simulink model "Lab7_E1"  (R2020b)
settings: Solver=VariableStepAuto  StartTime=0.0  StopTime=10  FixedStep=0  RelTol=1e-3
libraries: neural x28, simulink x2
(part 1 of 2)
settings Model: Creator=smsmt  LastModifiedBy=smsmt

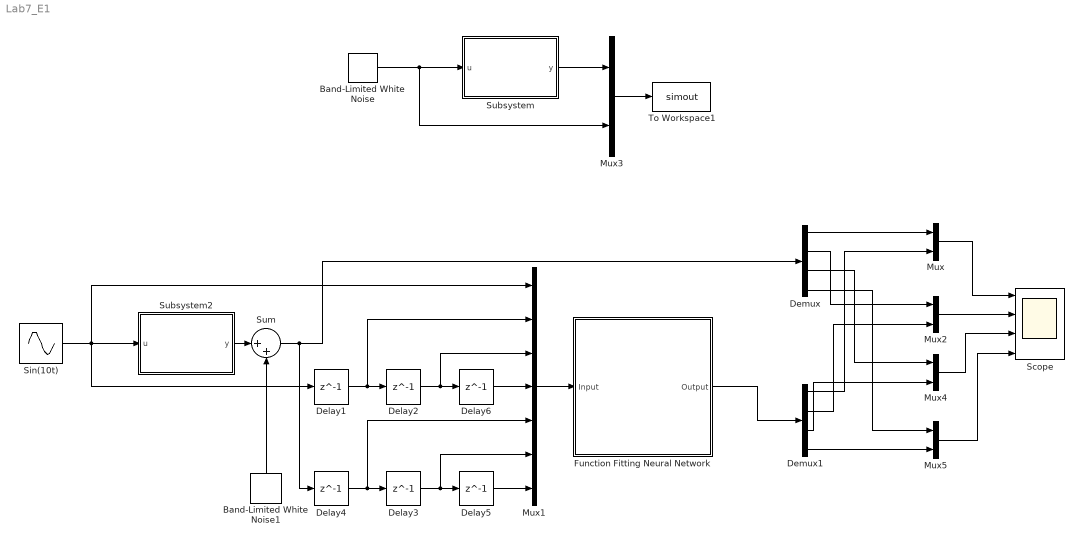
== system Lab7_E1 ==
  Band-Limited White Noise : simulink/Sources/Band-Limited White Noise  Cov=[0.1]  Ts=0.1  seed=[23341]
  Band-Limited White Noise1 : simulink/Sources/Band-Limited White Noise  Cov=[0.000]  Ts=0.1  seed=[23341]
  Delay{1..6} (6 alike) : Delay  DelayLength=1  InitialCondition=0
  Demux : Demux
  Demux1 : Demux
  Function Fitting Neural Network : Subsystem
      mask help: Function Fitting Neural Network
      mask Display: e = 0.06;c1 = [120 150 230]/255;c2 = ([120 150 230]+0)/383;c3 = ([120 150 230]+128)/383;patch([0 1 1 0],[0 0 1 1],c1);patch([0 1 1 1-e 1-e 0+e],[0 0 1 1-e 0+e 0+e],c2);patch([0 0 1 1-e 0+e 0+e],[0 1 1 1-e 1-e 0+e],c3);plot([0 1 1 0 0],[0 0 1 1 0]);fprintf('NNET');port_label('input',1,' Input');port_label('output',1,'Output ');
  Mux{,2..5} (5 alike) : Mux  Inputs=2
  Mux1 : Mux  Inputs=7
  Scope : Scope  NumInputPorts=4
  Sin(10t) : Sin  Frequency=10  SampleTime=0
  Subsystem : Subsystem
  Subsystem2 : Subsystem
  Sum : Sum  Inputs=|++
  To Workspace1 : ToWorkspace  VariableName=simout  SaveFormat=Timeseries  SampleTime=-1
  wires:
  Delay1/1 -> Mux1/2, Delay2/1
  Delay6/1 -> Mux1/4
  Delay4/1 -> Mux1/5, Delay3/1
  Mux1/1 -> Function Fitting Neural Network/1(Input)
  Delay5/1 -> Mux1/7
  Sin(10t)/1 -> Mux1/1, Delay1/1, Subsystem2/1(u)
  Subsystem2/1(y) -> Sum/1
  Delay2/1 -> Mux1/3, Delay6/1
  Delay3/1 -> Mux1/6, Delay5/1
  Mux3/1 -> To Workspace1/1
  Band-Limited White Noise/1 -> Subsystem/1(u), Mux3/2
  Subsystem/1(y) -> Mux3/1
  Function Fitting Neural Network/1(Output) -> Demux1/1
  Demux/1 -> Mux/1
  Demux1/1 -> Mux/2
  Mux/1 -> Scope/1
  Demux/2 -> Mux2/1
  Demux1/2 -> Mux2/2
  Demux/3 -> Mux4/1
  Demux1/3 -> Mux4/2
  Demux/4 -> Mux5/1
  Demux1/4 -> Mux5/2
  Mux5/1 -> Scope/4
  Mux4/1 -> Scope/3
  Mux2/1 -> Scope/2
  Sum/1 -> Delay4/1, Demux/1
  Band-Limited White Noise1/1 -> Sum/2

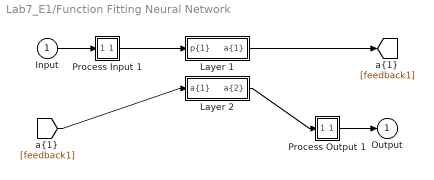
== system Lab7_E1/Function Fitting Neural Network ==
  Input : Inport  PortDimensions=16
      mask Display: e = 0.06;c1 = [120 230 180]/255;c2 = ([120 230 180]+0)/(256+128);c3 = ([120 230 180]+128)/(256+128);patch([0 1 1 0],[0 0 1 1],c1);patch([0 1 1 1-e 1-e 0+e],[0 0 1 1-e 0+e 0+e],c2);patch([0 0 1 1-e 0+e 0+e],[0 1 1 1-e 1-e 0+e],c3);plot([0 1 1 0 0],[0 0 1 1 0]);
  Layer 1 : Subsystem
      mask Display: e = 0.06;c1 = [120 150 230]/255;c2 = ([120 150 230]+0)/383;c3 = ([120 150 230]+128)/383;patch([0 1 1 0],[0 0 1 1],c1);patch([0 1 1 1-e 1-e 0+e],[0 0 1 1-e 0+e 0+e],c2);patch([0 0 1 1-e 0+e 0+e],[0 1 1 1-e 1-e 0+e],c3);plot([0 1 1 0 0],[0 0 1 1 0]);
  Layer 2 : Subsystem
      mask Display: e = 0.06;c1 = [120 150 230]/255;c2 = ([120 150 230]+0)/383;c3 = ([120 150 230]+128)/383;patch([0 1 1 0],[0 0 1 1],c1);patch([0 1 1 1-e 1-e 0+e],[0 0 1 1-e 0+e 0+e],c2);patch([0 0 1 1-e 0+e 0+e],[0 1 1 1-e 1-e 0+e],c3);plot([0 1 1 0 0],[0 0 1 1 0]);
  Process Input 1 : Subsystem
      mask Display: e = 0.06;c1 = [120 150 230]/255;c2 = ([120 150 230]+0)/383;c3 = ([120 150 230]+128)/383;patch([0 1 1 0],[0 0 1 1],c1);patch([0 1 1 1-e 1-e 0+e],[0 0 1 1-e 0+e 0+e],c2);patch([0 0 1 1-e 0+e 0+e],[0 1 1 1-e 1-e 0+e],c3);plot([0 1 1 0 0],[0 0 1 1 0]);
  Process Output 1 : Subsystem
      mask Display: e = 0.06;c1 = [120 150 230]/255;c2 = ([120 150 230]+0)/383;c3 = ([120 150 230]+128)/383;patch([0 1 1 0],[0 0 1 1],c1);patch([0 1 1 1-e 1-e 0+e],[0 0 1 1-e 0+e 0+e],c2);patch([0 0 1 1-e 0+e 0+e],[0 1 1 1-e 1-e 0+e],c3);plot([0 1 1 0 0],[0 0 1 1 0]);
  Output : Outport  InitialOutput=[0;0;0;0]
      mask Display: e = 0.06;c1 = [120 230 180]/255;c2 = ([120 230 180]+0)/(256+128);c3 = ([120 230 180]+128)/(256+128);patch([0 1 1 0],[0 0 1 1],c1);patch([0 1 1 1-e 1-e 0+e],[0 0 1 1-e 0+e 0+e],c2);patch([0 0 1 1-e 0+e 0+e],[0 1 1 1-e 1-e 0+e],c3);plot([0 1 1 0 0],[0 0 1 1 0]);
  wires:
  Input/1 -> Process Input 1/1(x)
  Process Output 1/1(y) -> Output/1
  Process Input 1/1(p) -> Layer 1/1("p{1}")
  Layer 1/1("a{1}") -> [feedback1]
  [feedback1] -> Layer 2/1("a{1} ")
  Layer 2/1("a{2}") -> Process Output 1/1(a)

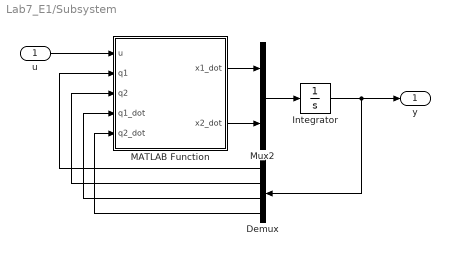
== system Lab7_E1/Subsystem ==
  u : Inport
  Demux : Demux
  Integrator : Integrator  InitialCondition=[0 0 0 0]
  MATLAB Function : MATLAB Function  TreatAsAtomicUnit=on
  Mux2 : Mux  Inputs=2
  y : Outport
  wires:
  Integrator/1 -> y/1, Demux/1
  u/1 -> MATLAB Function/1(u)
  MATLAB Function/1(x1_dot) -> Mux2/1
  MATLAB Function/2(x2_dot) -> Mux2/2
  Mux2/1 -> Integrator/1
  Demux/1 -> MATLAB Function/2(q1)
  Demux/2 -> MATLAB Function/3(q2)
  Demux/3 -> MATLAB Function/4(q1_dot)
  Demux/4 -> MATLAB Function/5(q2_dot)

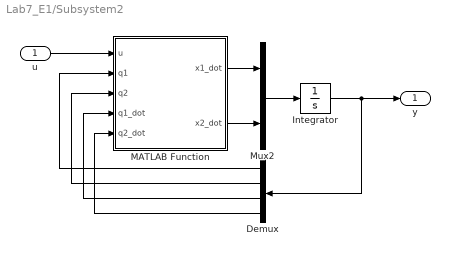
== system Lab7_E1/Subsystem2 ==
  u : Inport
  Demux : Demux
  Integrator : Integrator  InitialCondition=[0 0 0 0]
  MATLAB Function : MATLAB Function  TreatAsAtomicUnit=on
  Mux2 : Mux  Inputs=2
  y : Outport
  wires:
  Integrator/1 -> y/1, Demux/1
  u/1 -> MATLAB Function/1(u)
  MATLAB Function/1(x1_dot) -> Mux2/1
  MATLAB Function/2(x2_dot) -> Mux2/2
  Mux2/1 -> Integrator/1
  Demux/1 -> MATLAB Function/2(q1)
  Demux/2 -> MATLAB Function/3(q2)
  Demux/3 -> MATLAB Function/4(q1_dot)
  Demux/4 -> MATLAB Function/5(q2_dot)

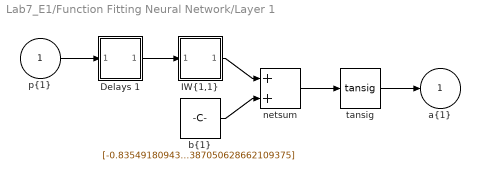
== system Lab7_E1/Function Fitting Neural Network/Layer 1 ==
  "p{1}" : Inport  PortDimensions=16
      mask Display: e = 0.06;c1 = [120 230 180]/255;c2 = ([120 230 180]+0)/(256+128);c3 = ([120 230 180]+128)/(256+128);patch([0 1 1 0],[0 0 1 1],c1);patch([0 1 1 1-e 1-e 0+e],[0 0 1 1-e 0+e 0+e],c2);patch([0 0 1 1-e 0+e 0+e],[0 1 1 1-e 1-e 0+e],c3);plot([0 1 1 0 0],[0 0 1 1 0]);
  Delays 1 : Subsystem
      mask Display: e = 0.06;c1 = [120 150 230]/255;c2 = ([120 150 230]+0)/383;c3 = ([120 150 230]+128)/383;patch([0 1 1 0],[0 0 1 1],c1);patch([0 1 1 1-e 1-e 0+e],[0 0 1 1-e 0+e 0+e],c2);patch([0 0 1 1-e 0+e 0+e],[0 1 1 1-e 1-e 0+e],c3);plot([0 1 1 0 0],[0 0 1 1 0]);disp('0');
  "IW{1,1}" : Subsystem
      mask Display: e = 0.06;c1 = [120 150 230]/255;c2 = ([120 150 230]+0)/383;c3 = ([120 150 230]+128)/383;patch([0 1 1 0],[0 0 1 1],c1);patch([0 1 1 1-e 1-e 0+e],[0 0 1 1-e 0+e 0+e],c2);patch([0 0 1 1-e 0+e 0+e],[0 1 1 1-e 1-e 0+e],c3);plot([0 1 1 0 0],[0 0 1 1 0]);disp('W');
  "b{1}" : Constant  Value=[-0.83549180943357848061481263357563875615596771240234375;-1.8201004242661380505552415343117900192737579345703125;0.92350959078641003952014898459310643374919891357421875;-0.92781891823089457371764865456498228013515472412109375;-0.98835326541109835840615005508880130946636199951171875;0.94440562253181947749425262372824363410472869873046875;-0.0199942887878296442216718986628620768897235393524169921875;-0.5282206006504706063964249551645480096340179443359375;-0.306513926556519933352973339424352161586284637451171875;0.00887448769022419238494681081874659867025911808013916015625;0.10503960517018810782996496300256694667041301727294921875;0.363930984793109202346528263660729862749576568603515625;0.853259192692973567062608708511106669902801513671875;-0.479073523910536536174475941152195446193218231201171875;0.386311529121468211211976040431181900203227996826171875;-0.50019372501267433950289387212251313030719757080078125;-0.84925071198815149653427170051145367324352264404296875;0.330688290295932219020613729298929683864116668701171875;1.0433757247374746413015600410290062427520751953125;1.810341107309246577727890326059423387050628662109375]
      mask Display: e = 0.06;c1 = [120 150 230]/255;c2 = ([120 150 230]+0)/383;c3 = ([120 150 230]+128)/383;patch([0 1 1 0],[0 0 1 1],c1);patch([0 1 1 1-e 1-e 0+e],[0 0 1 1-e 0+e 0+e],c2);patch([0 0 1 1-e 0+e 0+e],[0 1 1 1-e 1-e 0+e],c3);plot([0 1 1 0 0],[0 0 1 1 0]);disp('b');
  netsum : Sum  Inputs=2  InputSameDT=on  SaturateOnIntegerOverflow=on  OutDataTypeStr=Inherit: Same as first input
      mask Display: e = 0.06;c1 = [120 150 230]/255;c2 = ([120 150 230]+0)/383;c3 = ([120 150 230]+128)/383;patch([0 1 1 0],[0 0 1 1],c1);patch([0 1 1 1-e 1-e 0+e],[0 0 1 1-e 0+e 0+e],c2);patch([0 0 1 1-e 0+e 0+e],[0 1 1 1-e 1-e 0+e],c3);plot([0 1 1 0 0],[0 0 1 1 0]);disp('+');
  tansig : neural/Transfer Functions/tansig
  "a{1}" : Outport  InitialOutput=[0;0;0;0;0;0;0;0;0;0;0;0;0;0;0;0;0;0;0;0]
      mask Display: e = 0.06;c1 = [120 230 180]/255;c2 = ([120 230 180]+0)/(256+128);c3 = ([120 230 180]+128)/(256+128);patch([0 1 1 0],[0 0 1 1],c1);patch([0 1 1 1-e 1-e 0+e],[0 0 1 1-e 0+e 0+e],c2);patch([0 0 1 1-e 0+e 0+e],[0 1 1 1-e 1-e 0+e],c3);plot([0 1 1 0 0],[0 0 1 1 0]);
  wires:
  "p{1}"/1 -> Delays 1/1("p{1}")
  Delays 1/1("pd{1,1}") -> "IW{1,1}"/1("pd{1,1}")
  "IW{1,1}"/1("iz{1,1}") -> netsum/1
  "b{1}"/1 -> netsum/2
  netsum/1 -> tansig/1
  tansig/1 -> "a{1}"/1

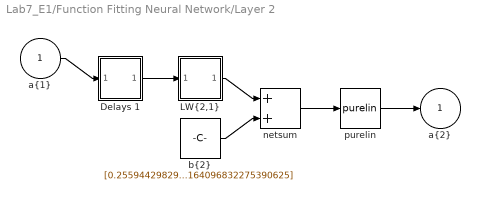
== system Lab7_E1/Function Fitting Neural Network/Layer 2 ==
  "a{1} " : Inport  PortDimensions=20
      mask Display: e = 0.06;c1 = [120 230 180]/255;c2 = ([120 230 180]+0)/(256+128);c3 = ([120 230 180]+128)/(256+128);patch([0 1 1 0],[0 0 1 1],c1);patch([0 1 1 1-e 1-e 0+e],[0 0 1 1-e 0+e 0+e],c2);patch([0 0 1 1-e 0+e 0+e],[0 1 1 1-e 1-e 0+e],c3);plot([0 1 1 0 0],[0 0 1 1 0]);
  Delays 1 : Subsystem
      mask Display: e = 0.06;c1 = [120 150 230]/255;c2 = ([120 150 230]+0)/383;c3 = ([120 150 230]+128)/383;patch([0 1 1 0],[0 0 1 1],c1);patch([0 1 1 1-e 1-e 0+e],[0 0 1 1-e 0+e 0+e],c2);patch([0 0 1 1-e 0+e 0+e],[0 1 1 1-e 1-e 0+e],c3);plot([0 1 1 0 0],[0 0 1 1 0]);disp('0');
  "LW{2,1}" : Subsystem
      mask Display: e = 0.06;c1 = [120 150 230]/255;c2 = ([120 150 230]+0)/383;c3 = ([120 150 230]+128)/383;patch([0 1 1 0],[0 0 1 1],c1);patch([0 1 1 1-e 1-e 0+e],[0 0 1 1-e 0+e 0+e],c2);patch([0 0 1 1-e 0+e 0+e],[0 1 1 1-e 1-e 0+e],c3);plot([0 1 1 0 0],[0 0 1 1 0]);disp('W');
  "b{2}" : Constant  Value=[0.25594429829992548786066208776901476085186004638671875;0.10194009318987629075792256116983480751514434814453125;0.55700857727010311126747410526149906218051910400390625;0.1142790231718998905652284747702651657164096832275390625]
      mask Display: e = 0.06;c1 = [120 150 230]/255;c2 = ([120 150 230]+0)/383;c3 = ([120 150 230]+128)/383;patch([0 1 1 0],[0 0 1 1],c1);patch([0 1 1 1-e 1-e 0+e],[0 0 1 1-e 0+e 0+e],c2);patch([0 0 1 1-e 0+e 0+e],[0 1 1 1-e 1-e 0+e],c3);plot([0 1 1 0 0],[0 0 1 1 0]);disp('b');
  netsum : Sum  Inputs=2  InputSameDT=on  SaturateOnIntegerOverflow=on  OutDataTypeStr=Inherit: Same as first input
      mask Display: e = 0.06;c1 = [120 150 230]/255;c2 = ([120 150 230]+0)/383;c3 = ([120 150 230]+128)/383;patch([0 1 1 0],[0 0 1 1],c1);patch([0 1 1 1-e 1-e 0+e],[0 0 1 1-e 0+e 0+e],c2);patch([0 0 1 1-e 0+e 0+e],[0 1 1 1-e 1-e 0+e],c3);plot([0 1 1 0 0],[0 0 1 1 0]);disp('+');
  purelin : neural/Transfer Functions/purelin
  "a{2}" : Outport  InitialOutput=[0;0;0;0]
      mask Display: e = 0.06;c1 = [120 230 180]/255;c2 = ([120 230 180]+0)/(256+128);c3 = ([120 230 180]+128)/(256+128);patch([0 1 1 0],[0 0 1 1],c1);patch([0 1 1 1-e 1-e 0+e],[0 0 1 1-e 0+e 0+e],c2);patch([0 0 1 1-e 0+e 0+e],[0 1 1 1-e 1-e 0+e],c3);plot([0 1 1 0 0],[0 0 1 1 0]);
  wires:
  "a{1} "/1 -> Delays 1/1("p{2}")
  Delays 1/1("pd{2,1}") -> "LW{2,1}"/1("ad{2,1}")
  "LW{2,1}"/1("lz{2,1}") -> netsum/1
  "b{2}"/1 -> netsum/2
  netsum/1 -> purelin/1
  purelin/1 -> "a{2}"/1

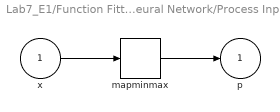
== system Lab7_E1/Function Fitting Neural Network/Process Input 1 ==
  x : Inport  PortDimensions=16
      mask Display: e = 0.06;c1 = [120 230 180]/255;c2 = ([120 230 180]+0)/(256+128);c3 = ([120 230 180]+128)/(256+128);patch([0 1 1 0],[0 0 1 1],c1);patch([0 1 1 1-e 1-e 0+e],[0 0 1 1-e 0+e 0+e],c2);patch([0 0 1 1-e 0+e 0+e],[0 1 1 1-e 1-e 0+e],c3);plot([0 1 1 0 0],[0 0 1 1 0]);
  mapminmax : neural/Processing Functions/mapminmax  xmin=[-3.60517824283159749043647934741;-3.60517824283159749043647934741;-3.60517824283159749043647934741;-3.60517824283159749043647934741;-3.14106589513792666679137255414;-0.492448062530743690956569480477;-2.84100174011369333015863958281;-0.745389047564771978215958370129;-3.14106589513792666679137255414;-0.492448062530743690956569480477;-2.84100174011369333015863958281;-0.745389047564771978215958370129;-3.14106589513792666679137255414;-0.492448062530743690956569480477;-2.84100174011369333015863958281;-0.745389047564771978215958370129]  xmax=[3.94389172900844897640126873739;3.94389172900844897640126873739;3.94389172900844897640126873739;3.94389172900844897640126873739;0.0005725595982868994515690985736;0.491232002437546833029102799628;2.83941327458839021247172240692;0.745062684061230662280195247149;0.0005725595982868994515690985736;0.491232002437546833029102799628;2.83941327458839021247172240692;0.745062684061230662280195247149;0.0005725595982868994515690985736;0.491232002437546833029102799628;2.83941327458839021247172240692;0.745062684061230662280195247149]  ymin=-1  ymax=1
  p : Outport  PortDimensions=16
      mask Display: e = 0.06;c1 = [120 230 180]/255;c2 = ([120 230 180]+0)/(256+128);c3 = ([120 230 180]+128)/(256+128);patch([0 1 1 0],[0 0 1 1],c1);patch([0 1 1 1-e 1-e 0+e],[0 0 1 1-e 0+e 0+e],c2);patch([0 0 1 1-e 0+e 0+e],[0 1 1 1-e 1-e 0+e],c3);plot([0 1 1 0 0],[0 0 1 1 0]);
  wires:
  x/1 -> mapminmax/1
  mapminmax/1 -> p/1

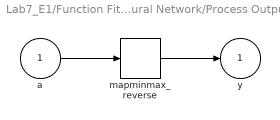
== system Lab7_E1/Function Fitting Neural Network/Process Output 1 ==
  a : Inport  PortDimensions=4
      mask Display: e = 0.06;c1 = [120 230 180]/255;c2 = ([120 230 180]+0)/(256+128);c3 = ([120 230 180]+128)/(256+128);patch([0 1 1 0],[0 0 1 1],c1);patch([0 1 1 1-e 1-e 0+e],[0 0 1 1-e 0+e 0+e],c2);patch([0 0 1 1-e 0+e 0+e],[0 1 1 1-e 1-e 0+e],c3);plot([0 1 1 0 0],[0 0 1 1 0]);
  mapminmax_reverse : neural/Processing Functions/mapminmax_reverse  xmin=[-3.14106589513792666679137255414;-0.492448062530743690956569480477;-2.84100174011369333015863958281;-0.745389047564771978215958370129]  xmax=[0.0005725595982868994515690985736;0.491232002437546833029102799628;2.83941327458839021247172240692;0.745062684061230662280195247149]  ymin=-1  ymax=1
  y : Outport  PortDimensions=4
      mask Display: e = 0.06;c1 = [120 230 180]/255;c2 = ([120 230 180]+0)/(256+128);c3 = ([120 230 180]+128)/(256+128);patch([0 1 1 0],[0 0 1 1],c1);patch([0 1 1 1-e 1-e 0+e],[0 0 1 1-e 0+e 0+e],c2);patch([0 0 1 1-e 0+e 0+e],[0 1 1 1-e 1-e 0+e],c3);plot([0 1 1 0 0],[0 0 1 1 0]);
  wires:
  a/1 -> mapminmax_reverse/1
  mapminmax_reverse/1 -> y/1

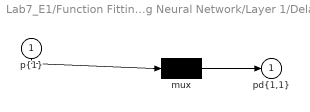
== system Lab7_E1/Function Fitting Neural Network/Layer 1/Delays 1 ==
  "p{1}" : Inport  PortDimensions=16
      mask Display: e = 0.06;c1 = [120 230 180]/255;c2 = ([120 230 180]+0)/(256+128);c3 = ([120 230 180]+128)/(256+128);patch([0 1 1 0],[0 0 1 1],c1);patch([0 1 1 1-e 1-e 0+e],[0 0 1 1-e 0+e 0+e],c2);patch([0 0 1 1-e 0+e 0+e],[0 1 1 1-e 1-e 0+e],c3);plot([0 1 1 0 0],[0 0 1 1 0]);
  mux : Mux  Inputs=1
      mask Display: e = 0.06;c1 = [120 150 230]/255;c2 = ([120 150 230]+0)/383;c3 = ([120 150 230]+128)/383;patch([0 1 1 0],[0 0 1 1],c1);patch([0 1 1 1-e 1-e 0+e],[0 0 1 1-e 0+e 0+e],c2);patch([0 0 1 1-e 0+e 0+e],[0 1 1 1-e 1-e 0+e],c3);plot([0 1 1 0 0],[0 0 1 1 0]);disp('Mux')
  "pd{1,1}" : Outport
      mask Display: e = 0.06;c1 = [120 230 180]/255;c2 = ([120 230 180]+0)/(256+128);c3 = ([120 230 180]+128)/(256+128);patch([0 1 1 0],[0 0 1 1],c1);patch([0 1 1 1-e 1-e 0+e],[0 0 1 1-e 0+e 0+e],c2);patch([0 0 1 1-e 0+e 0+e],[0 1 1 1-e 1-e 0+e],c3);plot([0 1 1 0 0],[0 0 1 1 0]);
  wires:
  "p{1}"/1 -> mux/1
  mux/1 -> "pd{1,1}"/1

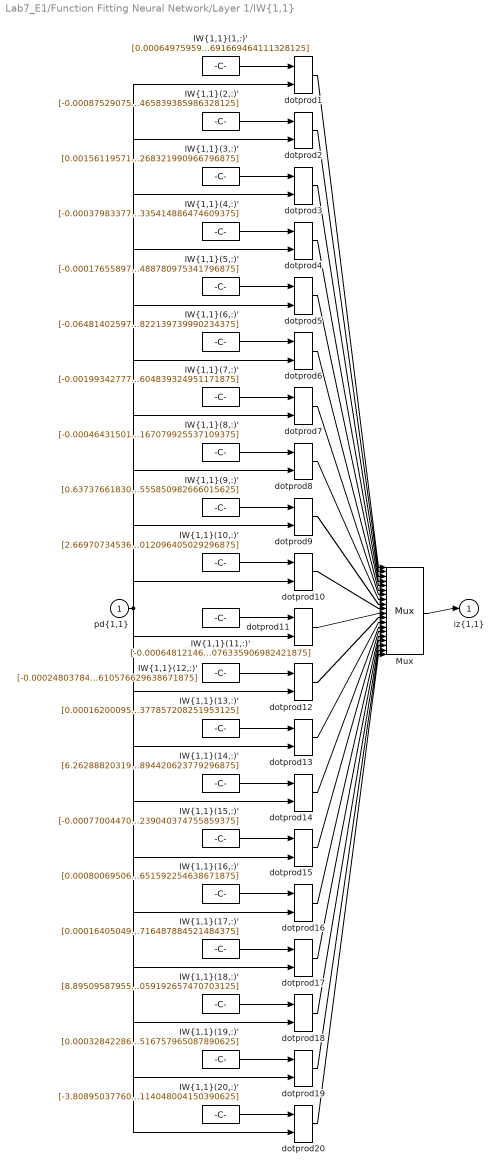
== system Lab7_E1/Function Fitting Neural Network/Layer 1/IW{1,1} ==
  "pd{1,1}" : Inport  PortDimensions=16
      mask Display: e = 0.06;c1 = [120 230 180]/255;c2 = ([120 230 180]+0)/(256+128);c3 = ([120 230 180]+128)/(256+128);patch([0 1 1 0],[0 0 1 1],c1);patch([0 1 1 1-e 1-e 0+e],[0 0 1 1-e 0+e 0+e],c2);patch([0 0 1 1-e 0+e 0+e],[0 1 1 1-e 1-e 0+e],c3);plot([0 1 1 0 0],[0 0 1 1 0]);
  "IW{1,1}(1,:)'" : Constant  Value=[0.0006497595962778571383744452560904392157681286334991455078125;-4.14681874647082770080248892430319074264843948185443878173828125e-05;-0.000117323732129381670869806841839277922190376557409763336181640625;-0.00081712479590169829861412420513033794122748076915740966796875;0.02054128798901501407048186820247792638838291168212890625;-0.222381987091993471583606378771946765482425689697265625;-0.08351944219501715449549550385199836455285549163818359375;-0.012355659297301264942792187184750218875706195831298828125;0.435902112701866517596727135241962969303131103515625;0.319137008096920304911492394239758141338825225830078125;0.1420357879260343292315837970818392932415008544921875;0.059008653478310912898763263001455925405025482177734375;-0.472592024618235073685212910277186892926692962646484375;-0.48057038845304023144677785239764489233493804931640625;-0.1660689221136188165051095211310894228518009185791015625;-0.1158794303381847357048428648340632207691669464111328125]
      mask Display: e = 0.06;c1 = [120 150 230]/255;c2 = ([120 150 230]+0)/383;c3 = ([120 150 230]+128)/383;patch([0 1 1 0],[0 0 1 1],c1);patch([0 1 1 1-e 1-e 0+e],[0 0 1 1-e 0+e 0+e],c2);patch([0 0 1 1-e 0+e 0+e],[0 1 1 1-e 1-e 0+e],c3);plot([0 1 1 0 0],[0 0 1 1 0]);disp('Weights');
  "IW{1,1}(10,:)'" : Constant  Value=[2.669707345365600827829556662695864588386029936373233795166015625e-05;6.163721756815836064040403652342092755134217441082000732421875e-05;0.00085904376332920592308772800294036642299033701419830322265625;-0.000748848611049175217659057413044365603127516806125640869140625;-0.64749101968490607728057284475653432309627532958984375;0.15628981793171414782506190022104419767856597900390625;0.41368487647578866539532782553578726947307586669921875;-0.25282757750305939747903494208003394305706024169921875;1.8245352517186936847082279200549237430095672607421875;-0.1258491512073245666147869314954732544720172882080078125;0.2105603075066311280494346647174097597599029541015625;0.39732536199083423600342257486772723495960235595703125;-1.1556706822333964179705390051822178065776824951171875;-0.0257373295222910851431930012722659739665687084197998046875;-0.441138402187714107061111690200050361454486846923828125;-0.17624767227669824176672364046680741012096405029296875]
      mask Display: e = 0.06;c1 = [120 150 230]/255;c2 = ([120 150 230]+0)/383;c3 = ([120 150 230]+128)/383;patch([0 1 1 0],[0 0 1 1],c1);patch([0 1 1 1-e 1-e 0+e],[0 0 1 1-e 0+e 0+e],c2);patch([0 0 1 1-e 0+e 0+e],[0 1 1 1-e 1-e 0+e],c3);plot([0 1 1 0 0],[0 0 1 1 0]);disp('Weights');
  "IW{1,1}(11,:)'" : Constant  Value=[-0.000648121461776643707948519779193929934990592300891876220703125;0.000318543579510111897479252007769900956191122531890869140625;0.00125256239143849818461207146214064778177998960018157958984375;-0.00020996056844432974962562366005869307628017850220203399658203125;-0.455149028189702098412539044147706590592861175537109375;0.0192023790503516693373153856327917310409247875213623046875;-0.202090650939533655883195706337573938071727752685546875;-0.1947404938538613572429625264703645370900630950927734375;0.314952753799047246996423154996591620147228240966796875;0.75358597806011273778636905262828804552555084228515625;0.002638631597796150911328094679220157559029757976531982421875;0.440502022320982344893991466960869729518890380859375;-0.2042047006275750364867604957908042706549167633056640625;-0.751880838415297514387702904059551656246185302734375;0.241867536319385789678193532381555996835231781005859375;-0.41794044873874092171917027371819131076335906982421875]
      mask Display: e = 0.06;c1 = [120 150 230]/255;c2 = ([120 150 230]+0)/383;c3 = ([120 150 230]+128)/383;patch([0 1 1 0],[0 0 1 1],c1);patch([0 1 1 1-e 1-e 0+e],[0 0 1 1-e 0+e 0+e],c2);patch([0 0 1 1-e 0+e 0+e],[0 1 1 1-e 1-e 0+e],c3);plot([0 1 1 0 0],[0 0 1 1 0]);disp('Weights');
  "IW{1,1}(12,:)'" : Constant  Value=[-0.0002480378412450206355131798741098236860125325620174407958984375;-0.00020751750405047168887735786757531286639277823269367218017578125;-0.00018989495924129386737223834646925979541265405714511871337890625;0.00034571509970268113516589369993425862048752605915069580078125;-0.11481098550833705729257161465284298174083232879638671875;-0.480672832578880993015246758659486658871173858642578125;0.2005000374408808239135026951771578751504421234130859375;0.00411778208916156567009903000098347547464072704315185546875;0.390440497022451704633994040705147199332714080810546875;0.465074648875374918599590046142111532390117645263671875;-0.5015642578297663245479043325758539140224456787109375;-0.09670273037684502803745800747492467053234577178955078125;-0.50558093037185580786996297320001758635044097900390625;-0.0940046176142029510369724221163778565824031829833984375;0.1497444992321221579612000596171128563582897186279296875;0.07308416151233614044269160103795002214610576629638671875]
      mask Display: e = 0.06;c1 = [120 150 230]/255;c2 = ([120 150 230]+0)/383;c3 = ([120 150 230]+128)/383;patch([0 1 1 0],[0 0 1 1],c1);patch([0 1 1 1-e 1-e 0+e],[0 0 1 1-e 0+e 0+e],c2);patch([0 0 1 1-e 0+e 0+e],[0 1 1 1-e 1-e 0+e],c3);plot([0 1 1 0 0],[0 0 1 1 0]);disp('Weights');
  "IW{1,1}(13,:)'" : Constant  Value=[0.00016200095803150493778931051647163030793308280408382415771484375;0.0003105684530270226323574178639574938642908819019794464111328125;0.000122863321462266385057648943046615386265330016613006591796875;-0.00124550561041928786569499276737360560218803584575653076171875;-0.1692623394344288378920992954590474255383014678955078125;-0.2970496022290927129461124422959983348846435546875;-0.0671470921687993549387130087779951281845569610595703125;0.1399743386114951915200066423494718037545680999755859375;0.50198259880397955168263024461339227855205535888671875;0.2158759395109148548907995746048982255160808563232421875;0.272103660620713616591359595986432395875453948974609375;0.29681257424949947232306612932006828486919403076171875;-0.153500660322007986824388581226230598986148834228515625;0.2078737494795244444834025898671825416386127471923828125;-0.0922669071525324124838363104572636075317859649658203125;-0.217394520222977949419629339899984188377857208251953125]
      mask Display: e = 0.06;c1 = [120 150 230]/255;c2 = ([120 150 230]+0)/383;c3 = ([120 150 230]+128)/383;patch([0 1 1 0],[0 0 1 1],c1);patch([0 1 1 1-e 1-e 0+e],[0 0 1 1-e 0+e 0+e],c2);patch([0 0 1 1-e 0+e 0+e],[0 1 1 1-e 1-e 0+e],c3);plot([0 1 1 0 0],[0 0 1 1 0]);disp('Weights');
  "IW{1,1}(14,:)'" : Constant  Value=[6.26288820319030928827908066836016587330959737300872802734375e-05;0.0003576643112834073582988192452347675498458556830883026123046875;-5.51893240529009778132414620888113176988554187119007110595703125e-05;-8.75221609081757064008133539800837752409279346466064453125e-05;0.779963663071746804433814759249798953533172607421875;0.2936522481223595715249530258006416261196136474609375;-0.418238868048481149397588296778849326074123382568359375;0.13467207616825771498980657270294614136219024658203125;-0.81612352358894046933102117691305465996265411376953125;-0.3477308428804641859954926985665224492549896240234375;0.2216233449633602525796760573939536698162555694580078125;-0.0309948291935520058026920509064439102075994014739990234375;-0.1869254427083924252617208594529074616730213165283203125;0.15814549301092772903842842424637638032436370849609375;-0.1390051880148988894259076687376364134252071380615234375;-0.0095404369545908467020733922936415183357894420623779296875]
      mask Display: e = 0.06;c1 = [120 150 230]/255;c2 = ([120 150 230]+0)/383;c3 = ([120 150 230]+128)/383;patch([0 1 1 0],[0 0 1 1],c1);patch([0 1 1 1-e 1-e 0+e],[0 0 1 1-e 0+e 0+e],c2);patch([0 0 1 1-e 0+e 0+e],[0 1 1 1-e 1-e 0+e],c3);plot([0 1 1 0 0],[0 0 1 1 0]);disp('Weights');
  "IW{1,1}(15,:)'" : Constant  Value=[-0.000770044701256342926758147182653146955999545753002166748046875;-0.000121153238827784843177626239452138179331086575984954833984375;0.000962624329641622732307848497868008053046651184558868408203125;0.001924798690870832031107884318998912931419909000396728515625;1.1900904568608223765835418817005120217800140380859375;-0.1664802091736500011531774134709849022328853607177734375;-0.68768212676038864561434138522599823772907257080078125;-0.250470894826118228859712644407409243285655975341796875;-1.3123900716313710024252259245258755981922149658203125;-0.26442442160472567902473883805214427411556243896484375;0.6451805147554383612629180788644589483737945556640625;-0.051426809903507501864350359710442717187106609344482421875;-0.03580352950115466004188391480056452564895153045654296875;0.294895585737153298477863927473663352429866790771484375;-0.200614027486274382194864074335782788693904876708984375;0.265400607909153762875575921498239040374755859375]
      mask Display: e = 0.06;c1 = [120 150 230]/255;c2 = ([120 150 230]+0)/383;c3 = ([120 150 230]+128)/383;patch([0 1 1 0],[0 0 1 1],c1);patch([0 1 1 1-e 1-e 0+e],[0 0 1 1-e 0+e 0+e],c2);patch([0 0 1 1-e 0+e 0+e],[0 1 1 1-e 1-e 0+e],c3);plot([0 1 1 0 0],[0 0 1 1 0]);disp('Weights');
  "IW{1,1}(16,:)'" : Constant  Value=[0.000800695062533548682602579926737007554038427770137786865234375;-0.00045715830620634352772502229100837212172336876392364501953125;0.0003268933807610846921203051618221024909871630370616912841796875;-5.997773816073786860326999548220783253782428801059722900390625e-05;-0.33597739810910909330488038904150016605854034423828125;0.267747073382606559643903665346442721784114837646484375;-0.57654563164647887330005460171378217637538909912109375;-0.334783999218468297787154597244807519018650054931640625;-0.2065178451448555774216941927079460583627223968505859375;-0.5471426101951986087357227006577886641025543212890625;-0.08439812068263206901175266239079064689576625823974609375;0.10666697974105117385779095684483763761818408966064453125;0.305545296852755388083977550195413641631603240966796875;0.262208114460602492723495515747345052659511566162109375;0.48284509012950216355619659225340001285076141357421875;0.1591205119241236587424026538428734056651592254638671875]
      mask Display: e = 0.06;c1 = [120 150 230]/255;c2 = ([120 150 230]+0)/383;c3 = ([120 150 230]+128)/383;patch([0 1 1 0],[0 0 1 1],c1);patch([0 1 1 1-e 1-e 0+e],[0 0 1 1-e 0+e 0+e],c2);patch([0 0 1 1-e 0+e 0+e],[0 1 1 1-e 1-e 0+e],c3);plot([0 1 1 0 0],[0 0 1 1 0]);disp('Weights');
  "IW{1,1}(17,:)'" : Constant  Value=[0.00016405049724810857707246736225670247222296893596649169921875;-0.0003472694094526647379771178147933596846996806561946868896484375;-0.000858663939336835814637727271048106558737345039844512939453125;1.745347316646612574326906386357194378433632664382457733154296875e-05;-1.669618756525871550167039458756335079669952392578125;-0.65396558716076125250538098043762147426605224609375;1.1620725576523589506194866771693341434001922607421875;0.07796620078256556729545678763315663672983646392822265625;1.3305314701478410110979666569619439542293548583984375;0.0988798833986821168462455489134299568831920623779296875;-1.2198542700796337623359022472868673503398895263671875;-0.0876473476984375443610275624450878240168094635009765625;0.481643337302925356180338667400064878165721893310546875;0.47629794668757530207159334167954511940479278564453125;0.538413625228424397306525861495174467563629150390625;0.08321182076209675260169973398660658858716487884521484375]
      mask Display: e = 0.06;c1 = [120 150 230]/255;c2 = ([120 150 230]+0)/383;c3 = ([120 150 230]+128)/383;patch([0 1 1 0],[0 0 1 1],c1);patch([0 1 1 1-e 1-e 0+e],[0 0 1 1-e 0+e 0+e],c2);patch([0 0 1 1-e 0+e 0+e],[0 1 1 1-e 1-e 0+e],c3);plot([0 1 1 0 0],[0 0 1 1 0]);disp('Weights');
  "IW{1,1}(18,:)'" : Constant  Value=[8.8950958795552698154564252863707451979280449450016021728515625e-05;0.00026509341560794594423733361310269174282439053058624267578125;-0.000403248729956397016470359684348068185499869287014007568359375;0.00142578383093951046971248342032367872889153659343719482421875;-1.3708659490516870160803364342427812516689300537109375;0.10422716158509580386404280716305947862565517425537109375;0.1593468523707887996021526078038732521235942840576171875;0.10771471872017539250787621085692080669105052947998046875;2.0941281483032572197089393739588558673858642578125;0.41506974766941018284427400431013666093349456787109375;0.053450916392035342783461970839198329485952854156494140625;-0.421772112283897160356360700461664237082004547119140625;-0.9212757175698806921815275927656330168247222900390625;-0.56291680190236392800073872422217391431331634521484375;0.0024612492798319189103717352651301553123630583286285400390625;0.26824387557028128714620152095449157059192657470703125]
      mask Display: e = 0.06;c1 = [120 150 230]/255;c2 = ([120 150 230]+0)/383;c3 = ([120 150 230]+128)/383;patch([0 1 1 0],[0 0 1 1],c1);patch([0 1 1 1-e 1-e 0+e],[0 0 1 1-e 0+e 0+e],c2);patch([0 0 1 1-e 0+e 0+e],[0 1 1 1-e 1-e 0+e],c3);plot([0 1 1 0 0],[0 0 1 1 0]);disp('Weights');
  "IW{1,1}(19,:)'" : Constant  Value=[0.000328422867463017630583477224348598610959015786647796630859375;-0.0004080776202633589204611663792121589722228236496448516845703125;-0.000170019236093398398192155784869328272179700434207916259765625;0.00015494386029386069607120812730016723435255698859691619873046875;-0.2088588702647231343245692869459162466228008270263671875;-0.55302265726755439612105647029238753020763397216796875;-0.0259466657331224419269499747997542726807296276092529296875;-0.10719727616281053694802238851480069570243358612060546875;0.08021692535129439083352309580732253380119800567626953125;0.326264227033478515505038330957177095115184783935546875;-0.493283374665843599160552912508137524127960205078125;-0.0419774265335615404115543469742988236248493194580078125;-0.322106224577082767002167429382097907364368438720703125;0.13030355446169694655367266022949479520320892333984375;0.177627801086429337740213441065861843526363372802734375;0.130231752558113422768570899279438890516757965087890625]
      mask Display: e = 0.06;c1 = [120 150 230]/255;c2 = ([120 150 230]+0)/383;c3 = ([120 150 230]+128)/383;patch([0 1 1 0],[0 0 1 1],c1);patch([0 1 1 1-e 1-e 0+e],[0 0 1 1-e 0+e 0+e],c2);patch([0 0 1 1-e 0+e 0+e],[0 1 1 1-e 1-e 0+e],c3);plot([0 1 1 0 0],[0 0 1 1 0]);disp('Weights');
  "IW{1,1}(2,:)'" : Constant  Value=[-0.000875290755914965852395315248912766037392430007457733154296875;0.0010655678861198150143840823744767476455308496952056884765625;0.002486375754704956385354730485914842574857175350189208984375;0.0028589814329637295610420100189230652176775038242340087890625;0.465150962009530155594205780289485119283199310302734375;0.0842845297424358597115912061781273223459720611572265625;0.463231932560459025438603930524550378322601318359375;-0.389883745641846191087864781366079114377498626708984375;-0.068338095445474589251233510367455892264842987060546875;-0.50530736805189813143357469016336835920810699462890625;-0.0312396333539726768491195940669058472849428653717041015625;0.2382435799123423236789420798231731168925762176513671875;-0.2963685885842635148179624593467451632022857666015625;0.330669736606570452419617822670261375606060028076171875;0.3546055544324790975707628604141063988208770751953125;0.363514908000529601839190263490309007465839385986328125]
      mask Display: e = 0.06;c1 = [120 150 230]/255;c2 = ([120 150 230]+0)/383;c3 = ([120 150 230]+128)/383;patch([0 1 1 0],[0 0 1 1],c1);patch([0 1 1 1-e 1-e 0+e],[0 0 1 1-e 0+e 0+e],c2);patch([0 0 1 1-e 0+e 0+e],[0 1 1 1-e 1-e 0+e],c3);plot([0 1 1 0 0],[0 0 1 1 0]);disp('Weights');
  "IW{1,1}(20,:)'" : Constant  Value=[-3.80895037760419334920032607971762672605109401047229766845703125e-05;-0.000714089892746204435436396806835546158254146575927734375;0.000678670392179360850749836320261465516523458063602447509765625;-0.00141509602233738239658589197489391153794713318347930908203125;-0.033249752747824157239620035397820174694061279296875;0.051727387772988277225838515960276708938181400299072265625;-0.7362248800639228374365075069363228976726531982421875;-0.25322434310274777313765071085072122514247894287109375;-0.0595268594475849843750125955921248532831668853759765625;0.47654820530768315922642841542256064713001251220703125;0.58005181467294131270051593673997558653354644775390625;0.291646757228084807511692133630276657640933990478515625;0.67851590896388158657970279818982817232608795166015625;-0.413777515725483435726772540874662809073925018310546875;-0.0767414846990561450024159739768947474658489227294921875;-0.27168882812889416644708262538188137114048004150390625]
      mask Display: e = 0.06;c1 = [120 150 230]/255;c2 = ([120 150 230]+0)/383;c3 = ([120 150 230]+128)/383;patch([0 1 1 0],[0 0 1 1],c1);patch([0 1 1 1-e 1-e 0+e],[0 0 1 1-e 0+e 0+e],c2);patch([0 0 1 1-e 0+e 0+e],[0 1 1 1-e 1-e 0+e],c3);plot([0 1 1 0 0],[0 0 1 1 0]);disp('Weights');
  "IW{1,1}(3,:)'" : Constant  Value=[0.00156119571766490518142933563439100907999090850353240966796875;0.0002498858016574074321532183962091266948846168816089630126953125;0.000627619329181742136199162462872891410370357334613800048828125;-0.0003498051026960557227489523324237552515114657580852508544921875;0.29474207246474259935808959198766387999057769775390625;-0.360346348681270856051384043894358910620212554931640625;-0.954539608379431303575302081299014389514923095703125;-0.03554218957472622675286544335904181934893131256103515625;-0.1991118793543983633842486824505613185465335845947265625;0.2365826967938474412189719942034571431577205657958984375;0.71750697359697579447157522736233659088611602783203125;0.23252378283572971984227706343517638742923736572265625;0.55771387205039413270668546829256229102611541748046875;0.411065088858833360685451907556853257119655609130859375;0.2479887610128704011902556203494896180927753448486328125;-0.00586174355902559056363809730783032136969268321990966796875]
      mask Display: e = 0.06;c1 = [120 150 230]/255;c2 = ([120 150 230]+0)/383;c3 = ([120 150 230]+128)/383;patch([0 1 1 0],[0 0 1 1],c1);patch([0 1 1 1-e 1-e 0+e],[0 0 1 1-e 0+e 0+e],c2);patch([0 0 1 1-e 0+e 0+e],[0 1 1 1-e 1-e 0+e],c3);plot([0 1 1 0 0],[0 0 1 1 0]);disp('Weights');
  "IW{1,1}(4,:)'" : Constant  Value=[-0.0003798337715813563633844573974585046016727574169635772705078125;-0.000249441646736257849337192737948498688638210296630859375;1.6775931835901871703488341669441297199227847158908843994140625e-05;0.0001929638547644634623441650678188352685538120567798614501953125;0.334971409197415581626700031847576610743999481201171875;0.1355361321430451349012713535557850264012813568115234375;0.122106224542132657528981098948861472308635711669921875;-0.11217024492258879930783876943678478710353374481201171875;-0.08147056444120910623230003011485678143799304962158203125;-0.5645243447692294136430746220867149531841278076171875;-0.5238313039339015375617236713878810405731201171875;-0.015808565293879063562432207845631637610495090484619140625;-0.7078430199216183549282277454040013253688812255859375;0.2850198232098872797024569081258960068225860595703125;0.05671871454815456681242125114295049570500850677490234375;0.0424693121194648914862312949480838142335414886474609375]
      mask Display: e = 0.06;c1 = [120 150 230]/255;c2 = ([120 150 230]+0)/383;c3 = ([120 150 230]+128)/383;patch([0 1 1 0],[0 0 1 1],c1);patch([0 1 1 1-e 1-e 0+e],[0 0 1 1-e 0+e 0+e],c2);patch([0 0 1 1-e 0+e 0+e],[0 1 1 1-e 1-e 0+e],c3);plot([0 1 1 0 0],[0 0 1 1 0]);disp('Weights');
  "IW{1,1}(5,:)'" : Constant  Value=[-0.00017655897202761079885224848595726143685169517993927001953125;-0.00055864550376499909171978952571180343511514365673065185546875;0.000973306377957160423312898966941020262311212718486785888671875;0.0002499754957638698348205974486546665502828545868396759033203125;0.32236641758659312362311766264610923826694488525390625;-0.345592372580953488547805818598135374486446380615234375;0.09845001681553029737603566218240302987396717071533203125;-0.459456519166919596930398483891622163355350494384765625;-0.5161355807762186831411099774413742125034332275390625;0.438490416258120296877365262844250537455081939697265625;0.0307753317906898603284471249708076356910169124603271484375;0.2670042013665305802305738325230777263641357421875;0.58171636948113081277966784909949637949466705322265625;-0.283880346642467973339307718561030924320220947265625;0.25123578453142070276982167342794127762317657470703125;0.007117496257319689927089978453977892058901488780975341796875]
      mask Display: e = 0.06;c1 = [120 150 230]/255;c2 = ([120 150 230]+0)/383;c3 = ([120 150 230]+128)/383;patch([0 1 1 0],[0 0 1 1],c1);patch([0 1 1 1-e 1-e 0+e],[0 0 1 1-e 0+e 0+e],c2);patch([0 0 1 1-e 0+e 0+e],[0 1 1 1-e 1-e 0+e],c3);plot([0 1 1 0 0],[0 0 1 1 0]);disp('Weights');
  "IW{1,1}(6,:)'" : Constant  Value=[-0.06481402597656064912268192301780800335109233856201171875;-0.004092143680449526928211145815339477849192917346954345703125;-0.0012426757535115950763227044006953292409889400005340576171875;0.03962134355508217797847692054347135126590728759765625;-0.5376738120341120197309692230192013084888458251953125;0.2078897200943762568758899078602553345263004302978515625;0.4602741249152708657987886908813379704952239990234375;-0.448534421738133903811984737330931238830089569091796875;-0.72057469504168825125134389963932335376739501953125;-0.323565035547536072879637458754586987197399139404296875;0.443999419790959415355047212869976647198200225830078125;0.497979192608943410647270866320468485355377197265625;0.07131032502471830458734558533251401968300342559814453125;-0.191349399559423150041226335815736092627048492431640625;-0.05783858737977214115044688469424727372825145721435546875;-0.8183361514022757798869633916183374822139739990234375]
      mask Display: e = 0.06;c1 = [120 150 230]/255;c2 = ([120 150 230]+0)/383;c3 = ([120 150 230]+128)/383;patch([0 1 1 0],[0 0 1 1],c1);patch([0 1 1 1-e 1-e 0+e],[0 0 1 1-e 0+e 0+e],c2);patch([0 0 1 1-e 0+e 0+e],[0 1 1 1-e 1-e 0+e],c3);plot([0 1 1 0 0],[0 0 1 1 0]);disp('Weights');
  "IW{1,1}(7,:)'" : Constant  Value=[-0.0019934277716382891622315387536445996374823153018951416015625;0.001158125043902765403946997224693404859863221645355224609375;0.00075377527919244058200731739560751520912162959575653076171875;0.002584609389924420741468935602824785746634006500244140625;-0.13675443197164816044875124134705401957035064697265625;-0.2045602257931095346865646433798247016966342926025390625;-0.743161918084098260806058533489704132080078125;0.1869992064266973452735243199640535749495029449462890625;0.245767995056967281097826116820215247571468353271484375;0.06897355358187196028296739314100705087184906005859375;0.77878189176789935910250051165348850190639495849609375;-0.26168055482685737000991821332718245685100555419921875;-0.36604073371679446413651248803944326937198638916015625;0.0238005007393906446722109393476785044185817241668701171875;-0.08538364482687736678467871342945727519690990447998046875;0.1587061194627694404868378796891192905604839324951171875]
      mask Display: e = 0.06;c1 = [120 150 230]/255;c2 = ([120 150 230]+0)/383;c3 = ([120 150 230]+128)/383;patch([0 1 1 0],[0 0 1 1],c1);patch([0 1 1 1-e 1-e 0+e],[0 0 1 1-e 0+e 0+e],c2);patch([0 0 1 1-e 0+e 0+e],[0 1 1 1-e 1-e 0+e],c3);plot([0 1 1 0 0],[0 0 1 1 0]);disp('Weights');
  "IW{1,1}(8,:)'" : Constant  Value=[-0.000464315012158815487719465409099939279258251190185546875;-5.50433352576753281613052004583863663356169126927852630615234375e-05;3.54743980116722037077177376307446365899522788822650909423828125e-05;0.000599036242651901557933202813188700019964016973972320556640625;-0.1665176304098157367139521056742523796856403350830078125;0.1723296329127926018731642443526652641594409942626953125;0.1143276934381814713415081996572553180158138275146484375;0.0026308882644641810866215081432528677396476268768310546875;0.462128128592325382317795856579323299229145050048828125;-0.0035193446620443223464558268887003578129224479198455810546875;-0.2303168440508232273078448315573041327297687530517578125;-0.0636182388528523656834323674047482199966907501220703125;-0.291272838800301914208290554597624577581882476806640625;0.12207777365622078658002891415890189819037914276123046875;0.1080157051453660976836346208074246533215045928955078125;0.073858481989838187242725098258233629167079925537109375]
      mask Display: e = 0.06;c1 = [120 150 230]/255;c2 = ([120 150 230]+0)/383;c3 = ([120 150 230]+128)/383;patch([0 1 1 0],[0 0 1 1],c1);patch([0 1 1 1-e 1-e 0+e],[0 0 1 1-e 0+e 0+e],c2);patch([0 0 1 1-e 0+e 0+e],[0 1 1 1-e 1-e 0+e],c3);plot([0 1 1 0 0],[0 0 1 1 0]);disp('Weights');
  "IW{1,1}(9,:)'" : Constant  Value=[0.63737661830385816674748866716981865465641021728515625;0.170284290525173409580617089886800386011600494384765625;0.279716443623468868917569807308609597384929656982421875;-0.38612799402853792418710554557037539780139923095703125;-0.25450926270260032513448322788462974131107330322265625;0.64598996345771386717871109794941730797290802001953125;-0.11904632672822124117573139301384799182415008544921875;0.017365618396402660028599029828910715878009796142578125;0.023192557068176362922162780932922032661736011505126953125;0.7427960376052828994630772285745479166507720947265625;0.31096415954111045198970941783045418560504913330078125;-0.2473609534895946093779883767638239078223705291748046875;-0.52745256211550028968559900022228248417377471923828125;-0.289909372803296261356109653206658549606800079345703125;0.4801704464988232334832218839437700808048248291015625;0.260223440899427116423936467981548048555850982666015625]
      mask Display: e = 0.06;c1 = [120 150 230]/255;c2 = ([120 150 230]+0)/383;c3 = ([120 150 230]+128)/383;patch([0 1 1 0],[0 0 1 1],c1);patch([0 1 1 1-e 1-e 0+e],[0 0 1 1-e 0+e 0+e],c2);patch([0 0 1 1-e 0+e 0+e],[0 1 1 1-e 1-e 0+e],c3);plot([0 1 1 0 0],[0 0 1 1 0]);disp('Weights');
  Mux : Mux  Inputs=20
      mask Display: e = 0.06;c1 = [120 150 230]/255;c2 = ([120 150 230]+0)/383;c3 = ([120 150 230]+128)/383;patch([0 1 1 0],[0 0 1 1],c1);patch([0 1 1 1-e 1-e 0+e],[0 0 1 1-e 0+e 0+e],c2);patch([0 0 1 1-e 0+e 0+e],[0 1 1 1-e 1-e 0+e],c3);plot([0 1 1 0 0],[0 0 1 1 0]);disp('Mux');
  dotprod{1..20} (20 alike) : neural/Weight Functions/dotprod
  "iz{1,1}" : Outport
      mask Display: e = 0.06;c1 = [120 230 180]/255;c2 = ([120 230 180]+0)/(256+128);c3 = ([120 230 180]+128)/(256+128);patch([0 1 1 0],[0 0 1 1],c1);patch([0 1 1 1-e 1-e 0+e],[0 0 1 1-e 0+e 0+e],c2);patch([0 0 1 1-e 0+e 0+e],[0 1 1 1-e 1-e 0+e],c3);plot([0 1 1 0 0],[0 0 1 1 0]);
  wires:
  "IW{1,1}(1,:)'"/1 -> dotprod1/1
  "pd{1,1}"/1 -> dotprod1/2, dotprod2/2, dotprod3/2, dotprod4/2, dotprod5/2, dotprod6/2, dotprod7/2, dotprod8/2, dotprod9/2, dotprod10/2, dotprod11/2, dotprod12/2, dotprod13/2, dotprod14/2, dotprod15/2, dotprod16/2, dotprod17/2, dotprod18/2, dotprod19/2, dotprod20/2
  dotprod1/1 -> Mux/1
  "IW{1,1}(2,:)'"/1 -> dotprod2/1
  dotprod2/1 -> Mux/2
  "IW{1,1}(3,:)'"/1 -> dotprod3/1
  dotprod3/1 -> Mux/3
  "IW{1,1}(4,:)'"/1 -> dotprod4/1
  dotprod4/1 -> Mux/4
  "IW{1,1}(5,:)'"/1 -> dotprod5/1
  dotprod5/1 -> Mux/5
  "IW{1,1}(6,:)'"/1 -> dotprod6/1
  dotprod6/1 -> Mux/6
  "IW{1,1}(7,:)'"/1 -> dotprod7/1
  dotprod7/1 -> Mux/7
  "IW{1,1}(8,:)'"/1 -> dotprod8/1
  dotprod8/1 -> Mux/8
  "IW{1,1}(9,:)'"/1 -> dotprod9/1
  dotprod9/1 -> Mux/9
  "IW{1,1}(10,:)'"/1 -> dotprod10/1
  dotprod10/1 -> Mux/10
  "IW{1,1}(11,:)'"/1 -> dotprod11/1
  dotprod11/1 -> Mux/11
  "IW{1,1}(12,:)'"/1 -> dotprod12/1
  dotprod12/1 -> Mux/12
  "IW{1,1}(13,:)'"/1 -> dotprod13/1
  dotprod13/1 -> Mux/13
  "IW{1,1}(14,:)'"/1 -> dotprod14/1
  dotprod14/1 -> Mux/14
  "IW{1,1}(15,:)'"/1 -> dotprod15/1
  dotprod15/1 -> Mux/15
  "IW{1,1}(16,:)'"/1 -> dotprod16/1
  dotprod16/1 -> Mux/16
  "IW{1,1}(17,:)'"/1 -> dotprod17/1
  dotprod17/1 -> Mux/17
  "IW{1,1}(18,:)'"/1 -> dotprod18/1
  dotprod18/1 -> Mux/18
  "IW{1,1}(19,:)'"/1 -> dotprod19/1
  dotprod19/1 -> Mux/19
  "IW{1,1}(20,:)'"/1 -> dotprod20/1
  dotprod20/1 -> Mux/20
  Mux/1 -> "iz{1,1}"/1

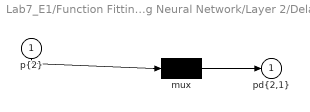
== system Lab7_E1/Function Fitting Neural Network/Layer 2/Delays 1 ==
  "p{2}" : Inport  PortDimensions=20
      mask Display: e = 0.06;c1 = [120 230 180]/255;c2 = ([120 230 180]+0)/(256+128);c3 = ([120 230 180]+128)/(256+128);patch([0 1 1 0],[0 0 1 1],c1);patch([0 1 1 1-e 1-e 0+e],[0 0 1 1-e 0+e 0+e],c2);patch([0 0 1 1-e 0+e 0+e],[0 1 1 1-e 1-e 0+e],c3);plot([0 1 1 0 0],[0 0 1 1 0]);
  mux : Mux  Inputs=1
      mask Display: e = 0.06;c1 = [120 150 230]/255;c2 = ([120 150 230]+0)/383;c3 = ([120 150 230]+128)/383;patch([0 1 1 0],[0 0 1 1],c1);patch([0 1 1 1-e 1-e 0+e],[0 0 1 1-e 0+e 0+e],c2);patch([0 0 1 1-e 0+e 0+e],[0 1 1 1-e 1-e 0+e],c3);plot([0 1 1 0 0],[0 0 1 1 0]);disp('Mux')
  "pd{2,1}" : Outport
      mask Display: e = 0.06;c1 = [120 230 180]/255;c2 = ([120 230 180]+0)/(256+128);c3 = ([120 230 180]+128)/(256+128);patch([0 1 1 0],[0 0 1 1],c1);patch([0 1 1 1-e 1-e 0+e],[0 0 1 1-e 0+e 0+e],c2);patch([0 0 1 1-e 0+e 0+e],[0 1 1 1-e 1-e 0+e],c3);plot([0 1 1 0 0],[0 0 1 1 0]);
  wires:
  "p{2}"/1 -> mux/1
  mux/1 -> "pd{2,1}"/1
